simulink model "trajetoria"  (R2022b)
settings: Solver=VariableStepAuto  StartTime=0.0  StopTime=10.0  RelTol=1e-3
settings Model: Creator=vfton  LastModifiedBy=matak
settings ModelReferenceCC: EnableRefExpFcnMdlSchedulingChecks=on

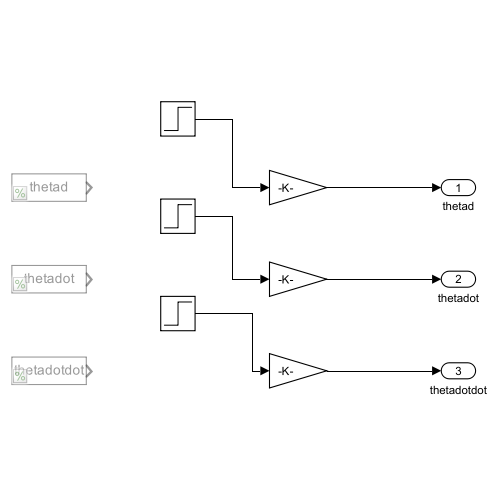
[thumbnail: Simulink's stored preview of the top-level diagram]
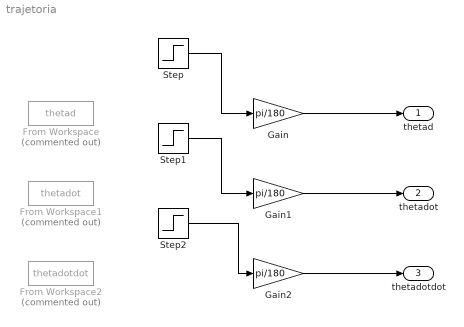
== system trajetoria ==
  From Workspace : FromWorkspace  Commented=on  VariableName=thetad  OutDataTypeStr=half
  From Workspace1 : FromWorkspace  Commented=on  VariableName=thetadot
  From Workspace2 : FromWorkspace  Commented=on  VariableName=thetadotdot
  Gain : Gain  Gain=pi/180
  Gain1 : Gain  Gain=pi/180
  Gain2 : Gain  Gain=pi/180
  Step : Step  Time=5  Before=[60; -110; 20]  After=[60; -50; 20]  SampleTime=0
  Step1 : Step  Time=20  Before=[0; 0; 0]  After=[0; 0; 0]  SampleTime=0
  Step2 : Step  Time=20  Before=[0; 0; 0]  After=[0; 0; 0]  SampleTime=0
  thetad : Outport
  thetadot : Outport  Port=2
  thetadotdot : Outport  Port=3
  wires:
  Gain/1 -> thetad/1
  Gain1/1 -> thetadot/1
  Gain2/1 -> thetadotdot/1
  Step/1 -> Gain/1
  Step1/1 -> Gain1/1
  Step2/1 -> Gain2/1
